simulink model "Vehicle_Model"  (R2022b)
settings: Solver=ode2  StartTime=T0  StopTime=Tf  FixedStep=Ts  EnableMultiTasking=on
model workspace (MAT data in the model file):
  aKalman : Simulink.Parameter (value not decoded)
  slipEnabler : Simulink.Parameter (value not decoded)
values from neighbouring files (symbols this model uses):
  enable_onlinePlots = 0    [main.m]
  enable_zoom = 1    [main.m]
  hv = 0.2    [main.m]
  lambda1_th = 0.1    [main.m]
  lambda2_th = 0.1    [main.m]
  LLC_sampleTime = LLC.sample_time    [main.m]
  longCTRparam = longitController()    [main.m]
  omega_LPF = 100    [main.m]
  previewPointParams = previewPointControllerParams()    [main.m]
  rho = 0.97    [main.m]
  rho_off = 0.9    [main.m]
  rho_on = 1.02    [main.m]
  road_data_sampled = [scenario_data.path.x_sampled', scenario_data.path.y_sampled']    [main.m]
  scenario_data = load(strcat('./Scenario/', scenario_name , '.mat'))    [main.m]
  T0 = scenario_data.times.t0    [main.m]
  tau_delta = vehicle_data.steering_system.tau_D    [main.m]
  Tb_dot_max = 5e3    (= 5000)    [main.m]
  Tb_max = 1000    [main.m]
  Tf = scenario_data.times.tf/2    [main.m]
  Ts = scenario_data.times.step_size    [main.m]
  v_on = 2.5    [main.m]
  v_stop = 0.1    [main.m]
  vehicle_data = getVehicleDataStruct()    [main.m]
  X0 = loadInitialConditions(scenario_data.vehicle_control.max_speed/3.6)    [main.m]
undefined symbols (not defined in the file or in its folder): DiscIntNeverNeededParam, latContr_select
libraries: simulink_extras x20, simulink x13, dspsigops x4, drivingvehiclecontroller x2, slpidlib x1
(part 2 of 2)

== system Vehicle_Model/Driver/Lateral Controller/Lateral Controller Clothoid-based ==
  targetPoint : Inport
  pose : Inport  Port=2
  speed : Inport  Port=3
  endOfCircuit : Inport  Port=4
  Action Port : ActionPort  ActionPortLabel=case [ 4 ]:
  MATLAB System : MATLABSystem  System=clothoidBased_lateralController  lookAhead=clothoidBasedParams.lookAhead  Kus=clothoidBasedParams.Kus  L=vehicle_data.vehicle.L  SimulateUsing=Interpreted execution
      mask Type: clothoidBased_lateralController
      mask Display:
      | disp('clothoidBased_lateralController');
      | port_label('input',1,'targetPoint');
      | port_label('input',2,'vehPose');
      | port_label('input',3,'vehSpeed');
      | port_label('input',4,'endOfCircuit');
      | port_label('output',1,'delta_req');
  Selector : Selector  InputPortWidth=4  IndexOptions=Index vector (dialog)  Indices=[1 2 3]  OutputSizes=1
  delta : Outport  VectorParamsAs1DForOutWhenUnconnected=off
  wires:
  speed/1 -> MATLAB System/3
  MATLAB System/1 -> delta/1
  pose/1 -> MATLAB System/2
  targetPoint/1 -> Selector/1
  Selector/1 -> MATLAB System/1
  endOfCircuit/1 -> MATLAB System/4

== system Vehicle_Model/Driver/Lateral Controller/Lateral Controller Stanley Dynamic ==
  targetPoint : Inport
  pose : Inport  Port=2
  speed : Inport  Port=3
  yaw_rate : Inport  Port=4
  steer_ang : Inport  Port=5
  Action Port : ActionPort  ActionPortLabel=case [ 3 ]:
  Constant : Constant
  Degrees to Radians : simulink_extras/Transformations/Degrees to Radians
  Helper Stanley Dynamic : MATLAB Function  TreatAsAtomicUnit=on
  Lateral Controller Stanley Dynamic : drivingvehiclecontroller/Lateral Controller Stanley  ModelType=Dynamic bicycle model  PositionGainF=stanleyParams.positGainFW  PositionGainR=stanleyParams.positGainREV  YawRateGain=stanleyParams.yawRateGain  DelayGain=stanleyParams.steerGain  VehicleMass=vehicle_data.vehicle.m  Lf=vehicle_data.vehicle.Lf  Lr=vehicle_data.vehicle.Lr  TireStiffness=stanleyParams.cornerStiff  Wheelbase=2.8  MaxSteeringAngle=stanleyParams.maxSteerAngle
  Radians to Degrees : simulink_extras/Transformations/Radians to Degrees
  Selector : Selector  InputPortWidth=4  IndexOptions=Index vector (dialog)  Indices=[1 2 3]  OutputSizes=1
  Selector1 : Selector  InputPortWidth=4  IndexOptions=Index vector (dialog)  Indices=[4]  OutputSizes=1
  delta : Outport  VectorParamsAs1DForOutWhenUnconnected=off
  wires:
  Lateral Controller Stanley Dynamic/1 -> Degrees to Radians/1
  pose/1 -> Helper Stanley Dynamic/1(pose)
  speed/1 -> Lateral Controller Stanley Dynamic/3
  Constant/1 -> Lateral Controller Stanley Dynamic/4
  Degrees to Radians/1 -> delta/1
  Helper Stanley Dynamic/1(currPose) -> Lateral Controller Stanley Dynamic/2
  targetPoint/1 -> Selector1/1, Selector/1
  Selector/1 -> Lateral Controller Stanley Dynamic/1
  Selector1/1 -> Lateral Controller Stanley Dynamic/5
  yaw_rate/1 -> Lateral Controller Stanley Dynamic/6
  Radians to Degrees/1 -> Lateral Controller Stanley Dynamic/7
  steer_ang/1 -> Radians to Degrees/1

== system Vehicle_Model/Driver/Lateral Controller/Lateral Controller Stanley Kinematic ==
  targetPoint : Inport
  pose : Inport  Port=2
  speed : Inport  Port=3
  Action Port : ActionPort  ActionPortLabel=case [ 2 ]:
  Constant : Constant
  Degrees to Radians : simulink_extras/Transformations/Degrees to Radians
  Helper Stanley Kinematic : MATLAB Function  TreatAsAtomicUnit=on
  Lateral Controller Stanley Kinematic : drivingvehiclecontroller/Lateral Controller Stanley  ModelType=Kinematic bicycle model  PositionGainF=stanleyParams.positGainFW  PositionGainR=stanleyParams.positGainREV  YawRateGain=0.2  DelayGain=0.2  VehicleMass=1575  Lf=1.2  Lr=1.6  TireStiffness=19000  Wheelbase=vehicle_data.vehicle.Lf + vehicle_data.vehicle.Lr  MaxSteeringAngle=stanleyParams.maxSteerAngle
  Selector : Selector  InputPortWidth=4  IndexOptions=Index vector (dialog)  Indices=[1 2 3]  OutputSizes=1
  delta : Outport  VectorParamsAs1DForOutWhenUnconnected=off
  wires:
  Lateral Controller Stanley Kinematic/1 -> Degrees to Radians/1
  pose/1 -> Helper Stanley Kinematic/1(pose)
  speed/1 -> Lateral Controller Stanley Kinematic/3
  Constant/1 -> Lateral Controller Stanley Kinematic/4
  Degrees to Radians/1 -> delta/1
  Helper Stanley Kinematic/1(currPose) -> Lateral Controller Stanley Kinematic/2
  targetPoint/1 -> Selector/1
  Selector/1 -> Lateral Controller Stanley Kinematic/1

== system Vehicle_Model/Driver/Lateral Controller/Preview point lateral Controller ==
  targetPoint : Inport
  endOfCircuit : Inport  Port=2
  Action Port : ActionPort  ActionPortLabel=case [ 5 ]:
  Constant : Constant  Value=previewPointParams.ke
  Constant1 : Constant  Value=previewPointParams.kp
  Preview Point Controller : MATLAB Function  TreatAsAtomicUnit=on
  delta : Outport  VectorParamsAs1DForOutWhenUnconnected=off
  wires:
  Preview Point Controller/1(delta) -> delta/1
  targetPoint/1 -> Preview Point Controller/1(target_Point)
  endOfCircuit/1 -> Preview Point Controller/4(endOfCircuit)
  Constant/1 -> Preview Point Controller/2(ke)
  Constant1/1 -> Preview Point Controller/3(kp)

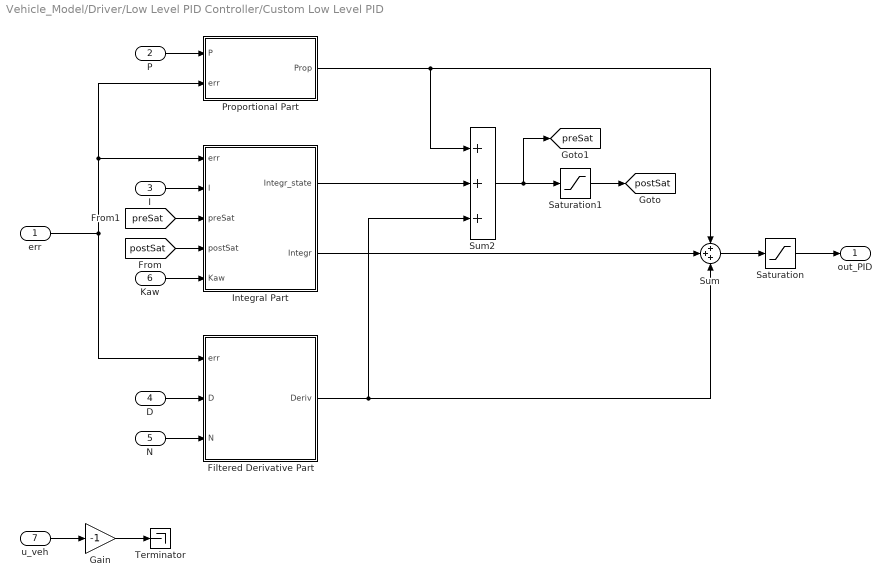
== system Vehicle_Model/Driver/Low Level PID Controller/Custom Low Level PID ==
  err : Inport
  P : Inport  Port=2
  I : Inport  Port=3
  D : Inport  Port=4
  N : Inport  Port=5
  Kaw : Inport  Port=6
  u_veh : Inport  Port=7
  Filtered Derivative Part : Subsystem
  Gain : Gain  Gain=-1
  Integral Part : Subsystem
  Proportional Part : Subsystem
  Saturation : Saturate  UpperLimit=1  LowerLimit=-1  LinearizeAsGain=off
  Saturation1 : Saturate  UpperLimit=1  LowerLimit=-1  LinearizeAsGain=off
  Sum : Sum  Inputs=+++
  Sum2 : Sum  Inputs=+++
  Terminator : Terminator
  out_PID : Outport  VectorParamsAs1DForOutWhenUnconnected=off
  tag scope: postSat=global, preSat=global
  wires:
  Sum2/1 -> [preSat], Saturation1/1
  Sum/1 -> Saturation/1
  Saturation/1 -> out_PID/1
  err/1 -> Filtered Derivative Part/1(err), Proportional Part/2(err), Integral Part/1(err)
  Saturation1/1 -> [postSat]
  I/1 -> Integral Part/2(I)
  Integral Part/1(Integr_state) -> Sum2/2
  Integral Part/2(Integr) -> Sum/2
  Proportional Part/1(Prop) -> Sum2/1, Sum/1
  P/1 -> Proportional Part/1(P)
  [preSat] -> Integral Part/3(preSat)
  [postSat] -> Integral Part/4(postSat)
  Filtered Derivative Part/1(Deriv) -> Sum/3, Sum2/3
  D/1 -> Filtered Derivative Part/2(D)
  N/1 -> Filtered Derivative Part/3(N)
  u_veh/1 -> Gain/1
  Gain/1 -> Terminator/1
  Kaw/1 -> Integral Part/5(Kaw)

== system Vehicle_Model/Driver/Low Level PID Controller/Custom Low Level PID/Filtered Derivative Part ==
  err : Inport
  D : Inport  Port=2
  N : Inport  Port=3
  Constant : Constant
  Discrete Transfer Fcn : DiscreteTransferFcn  Numerator=[1 -1]  DenominatorSource=Input port  SampleTime=Ts  a0EqualsOne=on
      settings: InputPortMap=u0,p3
  Gain1 : Gain  Gain=Ts/2
  Math Function : Math  Operator=reciprocal  SignedPower=on
  Mux1 : Mux  Inputs=2
  Product{2..5} (4 alike) : Product
  SumDen : Sum  Inputs=++|
  SumNum : Sum  Inputs=-+|
  Deriv : Outport  VectorParamsAs1DForOutWhenUnconnected=off
  wires:
  N/1 -> Gain1/1, Product5/2
  Product4/1 -> Product5/1
  SumDen/1 -> Math Function/1
  Math Function/1 -> Product4/2, Product3/1
  SumNum/1 -> Product3/2
  Product2/1 -> Discrete Transfer Fcn/1
  Discrete Transfer Fcn/1 -> Product4/1
  Constant/1 -> SumNum/1, SumDen/1, Mux1/1
  Product3/1 -> Mux1/2
  Mux1/1 -> Discrete Transfer Fcn/2
  Gain1/1 -> SumNum/2, SumDen/2
  err/1 -> Product2/1
  D/1 -> Product2/2
  Product5/1 -> Deriv/1

== system Vehicle_Model/Driver/Low Level PID Controller/Custom Low Level PID/Integral Part ==
  err : Inport
  I : Inport  Port=2
  preSat : Inport  Port=3
  postSat : Inport  Port=4
  Kaw : Inport  Port=5
  Anti-windup : Subsystem
  Discrete-Time Integrator1 : DiscreteIntegrator  IntegratorMethod=Integration: Trapezoidal  SampleTime=Ts  ShowStatePort=on  ICPrevOutput=DiscIntNeverNeededParam  ICPrevScaledInput=DiscIntNeverNeededParam
  Product1 : Product
  Integr_state : Outport  VectorParamsAs1DForOutWhenUnconnected=off
  Integr : Outport  Port=2  VectorParamsAs1DForOutWhenUnconnected=off
  wires:
  Discrete-Time Integrator1/State -> Integr_state/1
  preSat/1 -> Anti-windup/2(preSat)
  Product1/1 -> Anti-windup/4(preInt)
  postSat/1 -> Anti-windup/3(postSat)
  I/1 -> Product1/2
  Anti-windup/1(Out_antiWindUp) -> Discrete-Time Integrator1/1
  Discrete-Time Integrator1/1 -> Integr/1
  err/1 -> Product1/1
  Kaw/1 -> Anti-windup/1(Kaw)

== system Vehicle_Model/Driver/Low Level PID Controller/Custom Low Level PID/Proportional Part ==
  P : Inport
  err : Inport  Port=2
  Product : Product
  Prop : Outport  VectorParamsAs1DForOutWhenUnconnected=off
  wires:
  P/1 -> Product/2
  Product/1 -> Prop/1
  err/1 -> Product/1

== system Vehicle_Model/Driver/Low Level PID Controller/Custom Low Level PID/Integral Part/Anti-windup ==
  Kaw : Inport
  preSat : Inport  Port=2
  postSat : Inport  Port=3
  preInt : Inport  Port=4
  Product : Product
  Sum : Sum  Inputs=|-+
  Sum1 : Sum  Inputs=|++
  Out_antiWindUp : Outport  VectorParamsAs1DForOutWhenUnconnected=off
  wires:
  preSat/1 -> Sum/1
  preInt/1 -> Sum1/2
  Product/1 -> Sum1/1
  Sum1/1 -> Out_antiWindUp/1
  Sum/1 -> Product/2
  postSat/1 -> Sum/2
  Kaw/1 -> Product/1

== matlab function Vehicle_Model/Vehicle Model ==
  settings: sampleTime=step_size
  data: dX_prev input; X input; Tw__rr_brake input; Tw__rl_brake input; Tw__fr_brake input; Tw__fl_brake input; Tm_req input; dX output; extra_params output; delta_req input; vehicle_data parameter; road_condition input
function [dX,extra_params] = Vehicle_model(dX_prev,X,Tw__rr_brake,Tw__rl_brake,Tw__fr_brake,Tw__fl_brake,Tm_req,delta_req,vehicle_data,road_condition)

% ----------------------------------------------------------------
%% Double Track Vehicle Model
%  authors: 
%  rev. 1.0 Mattia Piccinini & Gastone Pietro Papini Rosati
%  rev. 2.0 Edoardo Pagot
%  date:
%  rev 1.0:    13/10/2020
%  rev 2.0:    16/05/2022
% ----------------------------------------------------------------


% ----------------------------------------------------------------
%% INPUTS OF THE MODEL
% ----------------------------------------------------------------

% Model inputs are: 
%       - requested wheel torques
%       - requested steering angle at the steering wheel delta_req (in [rad])


% ----------------------------------------------------------------
%% OUTPUTS OF THE MODEL
% ----------------------------------------------------------------

% The outputs of the model are the derivatives of all vehicle states,
% collected in the dX vector, as well as some other useful extra parameters 
% to describe vehicle behavior, saved in the extra_params vector

% Empty output vectors are here initialized 
dX = zeros(23,1);  
extra_params = zeros(23,1);  


% ----------------------------------------------------------------
%% STATES OF THE MODEL
% ----------------------------------------------------------------

x         = X(1);       % [m] x-coord of the vehicle CoM
y         = X(2);       % [m] x-coord of the vehicle CoM
psi       = X(3);       % [rad] yaw angle
u         = X(4);       % [m/s] vehicle longitudinal speed
v         = X(5);       % [m/s] vehicle lateral speed
Omega     = X(6);       % [rad/s] yaw rate
Fz__rr    = X(7);       % [N] vertical force for the rear right wheel
Fz__rl    = X(8);       % [N] vertical force for the rear left wheel
Fz__fr    = X(9);       % [N] vertical force for the front right wheel
Fz__fl    = X(10);      % [N] vertical force for the front left wheel
delta     = X(11);      % [rad] steering angle (at the wheel)
omega__rr = X(12);      % [rad/s] rotational speed rear right wheel
omega__rl = X(13);      % [rad/s] rotational speed rear left wheel 
omega__fr = X(14);      % [rad/s] rotational speed front right wheel 
omega__fl = X(15);      % [rad/s] rotational speed front left wheel 
alpha__rr = X(16);      % [rad] side slip angle rear right wheel
alpha__rl = X(17);      % [rad] side slip angle rear left wheel
alpha__fr = X(18);      % [rad] side slip angle front right wheel
alpha__fl = X(19);      % [rad] side slip angle front left wheel
kappa__rr = X(20);      % [-] longitudinal slip rear right wheel
kappa__rl = X(21);      % [-] longitudinal slip rear left wheel
kappa__fr = X(22);      % [-] longitudinal slip front right wheel
kappa__fl = X(23);      % [-] longitudinal slip front left wheel

% ----------------------------------------------------------------
%% AUXILIARY MODELS
% ----------------------------------------------------------------

% ----------------------
% MOTOR MODEL
% ----------------------
% Driving torques at the wheels
Tw__rr_traction = MotorModel(Tm_req,omega__rr,vehicle_data);
Tw__rl_traction = MotorModel(Tm_req,omega__rl,vehicle_data);

% Rear wheels braking model
Tw__rr_brake = brakeModelRear(Tw__rr_brake,omega__rr,vehicle_data); 
Tw__rl_brake = brakeModelRear(Tw__rl_brake,omega__rl,vehicle_data); 
% Front wheels braking model
Tw__fr_brake = brakeModelFront(Tw__fr_brake,omega__fr,vehicle_data);
Tw__fl_brake = brakeModelFront(Tw__fl_brake,omega__fl,vehicle_data);

% Total Torques
Tw__rr = Tw__rr_brake + Tw__rr_traction;
Tw__rl = Tw__rl_brake + Tw__rl_traction;
Tw__fr = Tw__fr_brake;
Tw__fl = Tw__fl_brake;


% ----------------------
% CAMBER MODEL
% ----------------------
[gamma__rr, gamma__rl, gamma__fr, gamma__fl] = camberModel(vehicle_data);

% ----------------------
% ACKERMANN STEERING MODEL
% ----------------------
% Compute steering angles for front wheels, with perfect Ackerman steering model
[delta__fr, delta__fl] = perfectAcker(delta,vehicle_data);

% ----------------------
% AERODYNAMIC MODEL
% ----------------------
% Aero drag, downforce at rear axle, downforce at front axle
[FAxc, FAz__r, FAz__f] = aeroModel(u,vehicle_data);

% ----------------------
% LONGITUDINAL SLIPS
% ----------------------
% Longitudinal slip model including a correction for low speed 
[kappa__rr_corr,kappa__rl_corr,kappa__fr_corr,kappa__fl_corr] = long_slip_low_speed(u,Omega,kappa__rr,kappa__rl,kappa__fr,kappa__fl,omega__rr,omega__rl,omega__fr,omega__fl,delta__fr,delta__fl,Fz__rr,Fz__rl,Fz__fr,Fz__fl,gamma__rr,gamma__rl,gamma__fr,gamma__fl,vehicle_data, road_condition);
          
% ----------------------
% ROAD CONDITION
% ----------------------
% Compute the aderenace of the asphalt 
road_condition_rr = road_condition(1);
road_condition_rl = road_condition(2);
road_condition_fr = road_condition(3);
road_condition_fl = road_condition(4);

% ----------------------
% TIRE PACEJKA MODEL
% ----------------------
% Ensure symmetric behavior of left and right tires by calculating the
% forces and moments for left tires via a previous change of sign of the
% side slip alpha and the camber gamma
% Side slip sign must be changed since data were fitted with reverse alpha
% sign

% RR
Fx__rr =  MF96_FX(kappa__rr_corr, -alpha__rr, -gamma__rr, Fz__rr, vehicle_data.tyre_data_r, road_condition_rr);
Fy__rr = -MF96_FY(kappa__rr_corr,  alpha__rr, -gamma__rr, Fz__rr, vehicle_data.tyre_data_r, road_condition_rr); % mirrored
AM__rr = -MF96_MZ(kappa__rr_corr,  alpha__rr, -gamma__rr, Fz__rr, vehicle_data.tyre_data_r, road_condition_rr); % mirrored

% RL
Fx__rl = MF96_FX(kappa__rl_corr, -alpha__rl, gamma__rl, Fz__rl, vehicle_data.tyre_data_r, road_condition_rl);
Fy__rl = MF96_FY(kappa__rl_corr, -alpha__rl, gamma__rl, Fz__rl, vehicle_data.tyre_data_r, road_condition_rl);
AM__rl = MF96_MZ(kappa__rl_corr, -alpha__rl, gamma__rl, Fz__rl, vehicle_data.tyre_data_r, road_condition_rl);

%FR
Fx__fr =  MF96_FX(kappa__fr_corr, -alpha__fr, -gamma__fr, Fz__fr, vehicle_data.tyre_data_f, road_condition_fr);
Fy__fr = -MF96_FY(kappa__fr_corr,  alpha__fr, -gamma__fr, Fz__fr, vehicle_data.tyre_data_f, road_condition_fr); % mirrored
AM__fr = -MF96_MZ(kappa__fr_corr,  alpha__fr, -gamma__fr, Fz__fr, vehicle_data.tyre_data_f, road_condition_fr); % mirrored

% FL
Fx__fl = MF96_FX(kappa__fl_corr, -alpha__fl, gamma__fl, Fz__fl, vehicle_data.tyre_data_f, road_condition_fl);
Fy__fl = MF96_FY(kappa__fl_corr, -alpha__fl, gamma__fl, Fz__fl, vehicle_data.tyre_data_f, road_condition_fl);
AM__fl = MF96_MZ(kappa__fl_corr, -alpha__fl, gamma__fl, Fz__fl, vehicle_data.tyre_data_f, road_condition_fl);


Mz_tires.rr = AM__rr;  Mz_tires.rl = AM__rl;  Mz_tires.fr = AM__fr;  Mz_tires.fl = AM__fl;

% ----------------------
% VERTICAL TIRE FORCES MODEL
% ----------------------
% Compute vertical tire loads
u_dot = dX_prev(4);
VerticalForces = LoadTransferModel(Omega,u,u_dot,FAz__r,FAz__f,Mz_tires,vehicle_data);
Fz__rr__ss = VerticalForces.Fz_rr_ss;
Fz__rl__ss = VerticalForces.Fz_rl_ss;
Fz__fr__ss = VerticalForces.Fz_fr_ss;
Fz__fl__ss = VerticalForces.Fz_fl_ss;

% ----------------------
% AXLE FORCES
% ----------------------
Fx__r = Fx__rr + Fx__rl;
Fx__f = Fx__fl - sin(delta__fl)*Fy__fl + Fx__fr - sin(delta__fr)*Fy__fr;
Fy__r = Fy__rl + Fy__rr;
Fy__f = sin(delta__fl)*Fx__fl + Fy__fl + sin(delta__fr)*Fx__fr + Fy__fr;
Delta__Fx__r = (Fx__rr-Fx__rl)/2;
Delta__Fx__f = ((Fx__fr - sin(delta__fr)*Fy__fr) - (Fx__fl - sin(delta__fl)*Fy__fl))/2;


% ----------------------
% STEADY STATE SLIPS
% ----------------------
% Longitudinal Slips
[kappa__rr__ss,kappa__rl__ss,kappa__fr__ss,kappa__fl__ss] = steadyStateLongSlips(omega__rr,omega__rl,omega__fr,omega__fl,Omega,u,delta__fr,delta__fl,vehicle_data);
% Lateral Slips
[alpha__rr__ss,alpha__rl__ss,alpha__fr__ss,alpha__fl__ss] = steadyStateLatSlips(Omega,u,v,delta__fr,delta__fl,vehicle_data);


% ----------------------------------------------------------------
%% VEHICLE DATA
% ----------------------------------------------------------------
m      = vehicle_data.vehicle.m;
Lf     = vehicle_data.vehicle.Lf;
Lr     = vehicle_data.vehicle.Lr;
Wf     = vehicle_data.vehicle.Wf;
Wr     = vehicle_data.vehicle.Wr;
izz    = vehicle_data.vehicle.i_zz;
tau__N = vehicle_data.suspension.tau_N;
tau__D = vehicle_data.steering_system.tau_D;
tau__H = vehicle_data.steering_system.tau_H;
ly     = vehicle_data.vehicle.ly;
lx     = vehicle_data.vehicle.lx;
iwa__r = vehicle_data.rear_wheel.iwa_r;
iwa__f = vehicle_data.front_wheel.iwa_f;
Rr     = vehicle_data.rear_wheel.Rr;
Rf     = vehicle_data.front_wheel.Rf;

% ----------------------------------------------------------------
%% VEHICLE MODEL DIFFERENTIAL EQUATIONS
% ----------------------------------------------------------------

% The following system of ODE is imported from Maple symbolic model

% Evolution of vehicle pose
x_dot        = u*cos(psi) - v*sin(psi);
y_dot        = v*cos(psi) + u*sin(psi);
psi_dot      = Omega;
% Newton equations
u_Dot        = (Omega * m * v - FAxc + Fx__f + Fx__r) / m;
v_Dot        = (-Omega * m * u + Fy__f + Fy__r) / m;
% Euler equation
Omega_Dot    = (Lf * Fy__f - Lr * Fy__r + Wf * Delta__Fx__f + Wr * Delta__Fx__r + AM__fl + AM__fr + AM__rl + AM__rr) / izz;
% Vertical loads first order dynamics
Fz_rr_Dot    = (-Fz__rr + Fz__rr__ss) / tau__N;
Fz_rl_Dot    = (-Fz__rl + Fz__rl__ss) / tau__N;
Fz_fr_Dot    = (-Fz__fr + Fz__fr__ss) / tau__N;
Fz_fl_Dot    = (-Fz__fl + Fz__fl__ss) / tau__N;
% Steering wheel first order dynamics
delta_Dot    = (-delta * tau__D + delta_req) / tau__D / tau__H;
% Side slip angle first order dynamics
alpha_rr_Dot = -(alpha__rr - alpha__rr__ss) * abs(u) / ly;
alpha_rl_Dot = -(alpha__rl - alpha__rl__ss) * abs(u) / ly;
alpha_fr_Dot = -(alpha__fr - alpha__fr__ss) * abs(u) / ly;
alpha_fl_Dot = -(alpha__fl - alpha__fl__ss) * abs(u) / ly;
% Longitudinal slip first order dynamics
kappa_rr_Dot = -abs(u) * (kappa__rr - kappa__rr__ss) / lx;
kappa_rl_Dot = -abs(u) * (kappa__rl - kappa__rl__ss) / lx;
kappa_fr_Dot = -abs(u) * (kappa__fr - kappa__fr__ss) / lx;
kappa_fl_Dot = -abs(u) * (kappa__fl - kappa__fl__ss) / lx;
% Wheel spin dynamics
omega_rr_Dot = (-Fx__rr * Rr + Tw__rr) / iwa__r;
omega_rl_Dot = (-Fx__rl * Rr + Tw__rl) / iwa__r;
omega_fr_Dot = (-Fx__fr * Rf + Tw__fr) / iwa__f;
omega_fl_Dot = (-Fx__fl * Rf + Tw__fl) / iwa__f;

% Collect states derivatives in the dX vector
dX(1)  = x_dot;
dX(2)  = y_dot;
dX(3)  = psi_dot;
dX(4)  = u_Dot;
dX(5)  = v_Dot;
dX(6)  = Omega_Dot;
dX(7)  = Fz_rr_Dot;
dX(8)  = Fz_rl_Dot;
dX(9)  = Fz_fr_Dot;
dX(10) = Fz_fl_Dot;
dX(11) = delta_Dot;
dX(12) = omega_rr_Dot;
dX(13) = omega_rl_Dot;
dX(14) = omega_fr_Dot;
dX(15) = omega_fl_Dot;
dX(16) = alpha_rr_Dot;
dX(17) = alpha_rl_Dot;
dX(18) = alpha_fr_Dot;
dX(19) = alpha_fl_Dot;
dX(20) = kappa_rr_Dot;
dX(21) = kappa_rl_Dot;
dX(22) = kappa_fr_Dot;
dX(23) = kappa_fl_Dot;


% ----------------------------------------------------------------
%% SAVE USEFUL EXTRA PARAMETERS
% ----------------------------------------------------------------

extra_params(1)  = Tw__rr;
extra_params(2)  = Tw__rl;
extra_params(3)  = Tw__fr;
extra_params(4)  = Tw__fl;
extra_params(5)  = Fx__rr;
extra_params(6)  = Fx__rl;
extra_params(7)  = Fx__fr;
extra_params(8)  = Fx__fl;
extra_params(9)  = Fy__rr;
extra_params(10) = Fy__rl;
extra_params(11) = Fy__fr;
extra_params(12) = Fy__fl;
extra_params(13) = AM__rr;
extra_params(14) = AM__rl;
extra_params(15) = AM__fr;
extra_params(16) = AM__fl;
extra_params(17) = gamma__rr;
extra_params(18) = gamma__rl;
extra_params(19) = gamma__fr;
extra_params(20) = gamma__fl;
extra_params(21) = delta__fr;
extra_params(22) = delta__fl;
extra_params(23) = delta_req;

end

== matlab function Vehicle_Model/ABS and Wheel torque generation/ABS Rear Right Wheel1/compute lambda ==
  data: u input; lambda output; omega input; vehicle_data parameter
function lambda = compute_lambda(u, omega, vehicle_data)

lambda = (u - omega*vehicle_data.rear_wheel.Rr)/u;

== stateflow chart Vehicle_Model/ABS and Wheel torque generation/ABS Rear Left Wheel1/Antilock Braking System/Activation and Deactivation Logic ==
  state abs_OFF
    ABS_ON = 0;
    state High_Speed_OFF
      Tb_select = 1;
    state Low_Speed_OFF
      Tb_select = 1;
    (default) -> High_Speed_OFF
    High_Speed_OFF -> Low_Speed_OFF [order 2] : [v < v_on - hv]
    Low_Speed_OFF -> High_Speed_OFF : [v > v_on + hv]
  state abs_ON
    ABS_ON = 1;
    state High_Speed_ON
      Tb_select = 2;
    state Low_Speed_ON
      Tb_select = 3;
    High_Speed_ON -> Low_Speed_ON [order 2] : [v < v_on]
  (default) -> abs_OFF
  High_Speed_OFF -> High_Speed_ON [order 1] : [v > v_on && ...
      | Tb_Dr > rho_on * Tb_Ctrl && ...
      | lambda > lambda1_th - (((lambda1_th - lambda2_th) * Tb_dot) / Tb_dot_max) ]
  High_Speed_ON -> High_Speed_OFF [order 1] : [Tb_Dr < rho_off * Tb_Ctrl]
  Low_Speed_ON -> Low_Speed_OFF : [v < v_stop || ...
      | Tb_Dr < rho_off * Tb_LPF]
  data: Tb_select output; Tb_Dr input; Tb_Ctrl input; v input; Tb_dot input; Tb_dot_max parameter; v_on parameter; rho_on parameter; Tb_LPF input; lambda input; lambda1_th parameter; v_stop parameter; hv parameter; rho_off parameter; ABS_ON output; lambda2_th parameter

== matlab function Vehicle_Model/ABS and Wheel torque generation/ABS Rear Left Wheel1/compute lambda ==
  data: u input; lambda output; omega input; vehicle_data parameter
function lambda = compute_lambda(u, omega, vehicle_data)

lambda = (u - omega*vehicle_data.rear_wheel.Rr)/u;

== stateflow chart Vehicle_Model/ABS and Wheel torque generation/ABS Front Right Wheel1/Antilock Braking System/Activation and Deactivation Logic ==
  state abs_OFF
    ABS_ON = 0;
    state High_Speed_OFF
      Tb_select = 1;
    state Low_Speed_OFF
      Tb_select = 1;
    (default) -> High_Speed_OFF
    High_Speed_OFF -> Low_Speed_OFF [order 2] : [v < v_on - hv]
    Low_Speed_OFF -> High_Speed_OFF : [v > v_on + hv]
  state abs_ON
    ABS_ON = 1;
    state High_Speed_ON
      Tb_select = 2;
    state Low_Speed_ON
      Tb_select = 3;
    High_Speed_ON -> Low_Speed_ON [order 2] : [v < v_on]
  (default) -> abs_OFF
  High_Speed_OFF -> High_Speed_ON [order 1] : [v > v_on && ...
      | Tb_Dr > rho_on * Tb_Ctrl && ...
      | lambda > lambda1_th - (((lambda1_th - lambda2_th) * Tb_dot) / Tb_dot_max) ]
  High_Speed_ON -> High_Speed_OFF [order 1] : [Tb_Dr < rho_off * Tb_Ctrl]
  Low_Speed_ON -> Low_Speed_OFF : [v < v_stop || ...
      | Tb_Dr < rho_off * Tb_LPF]
  data: Tb_select output; Tb_Dr input; Tb_Ctrl input; v input; Tb_dot input; Tb_dot_max parameter; v_on parameter; rho_on parameter; Tb_LPF input; lambda input; lambda1_th parameter; v_stop parameter; hv parameter; rho_off parameter; ABS_ON output; lambda2_th parameter

== matlab function Vehicle_Model/ABS and Wheel torque generation/ABS Front Right Wheel1/compute lambda ==
  data: u input; lambda output; omega input; vehicle_data parameter
function lambda = compute_lambda(u, omega, vehicle_data)

lambda = (u - omega*vehicle_data.rear_wheel.Rr)/u;

== matlab function Vehicle_Model/Estimate pose/Online Trajectory Plots/Plot manager ==
  data: vehiclePose input; targetPoint_steerCtrl input; enable_zoomMPC input; refPath input; latContr_type input
function real_time_plot(vehiclePose,targetPoint_steerCtrl,enable_zoomMPC,refPath,latContr_type)
    
    coder.extrinsic('patch');
    
    %% Extract vehicle pose
    xCoMCar = vehiclePose(1);
    yCoMCar = vehiclePose(2);
    vehicleAttitude = vehiclePose(3);
    
    %% Load vehicle data
    vehicle_data = getVehicleDataStruct();
    Lf = vehicle_data.vehicle.Lf;        
    Lr = vehicle_data.vehicle.Lr;                 
    Wf = vehicle_data.vehicle.Wf;     
    Wr = vehicle_data.vehicle.Wr;
    
    %% Delete the plots for the previous iteration
    cla;
    
    %% Sketch the vehicle and its position, for this MPC iteration
    % Rotation matrix from vehicle (mobile) frame to the absolute frame
    RotMat = [cos(vehicleAttitude), -sin(vehicleAttitude); ...
              sin(vehicleAttitude), cos(vehicleAttitude)];
    
    pos_vehRR = RotMat*[-Lr -Wr/2]';
    pos_vehRL = RotMat*[-Lr +Wr/2]';
    pos_vehFR = RotMat*[+Lf -Wf/2]';
    pos_vehFL = RotMat*[+Lf +Wf/2]';
    pos_veh   = [pos_vehRR pos_vehRL pos_vehFL pos_vehFR];
    
    % Optimal route computed with route planner
    X_route = refPath(:,1);
    Y_route = refPath(:,2);
    plot(X_route,Y_route,'go','MarkerSize',2)
    
    % Current vehicle pose
    patch(xCoMCar + pos_veh(1,:),yCoMCar + pos_veh(2,:),'yellow');
    
    % Objects of the road scenario (walls, fixed obstacles etc)
%     for ii=1:size(mapObjects,1)
%         rectangle('Position',mapObjects(ii,:),'FaceColor',color('purple'),'EdgeColor',color('purple'),'LineWidth',2)
%     end
    
    % Target point used by some low-level lateral controllers
    if (latContr_type==1 || latContr_type==4)  
        plot(targetPoint_steerCtrl(1),targetPoint_steerCtrl(2),'r*','MarkerSize',6)
    end
    
    % Zoom on the vehicle if required
    if (enable_zoomMPC)
        xlim([xCoMCar-40 xCoMCar+40])
        ylim([yCoMCar-40 yCoMCar+40])
    end
    
end

== stateflow chart Vehicle_Model/ABS and Wheel torque generation/ABS Front Left Wheel1/Antilock Braking System/Activation and Deactivation Logic ==
  state abs_OFF
    ABS_ON = 0;
    state High_Speed_OFF
      Tb_select = 1;
    state Low_Speed_OFF
      Tb_select = 1;
    (default) -> High_Speed_OFF
    High_Speed_OFF -> Low_Speed_OFF [order 2] : [v < v_on - hv]
    Low_Speed_OFF -> High_Speed_OFF : [v > v_on + hv]
  state abs_ON
    ABS_ON = 1;
    state High_Speed_ON
      Tb_select = 2;
    state Low_Speed_ON
      Tb_select = 3;
    High_Speed_ON -> Low_Speed_ON [order 2] : [v < v_on]
  (default) -> abs_OFF
  High_Speed_OFF -> High_Speed_ON [order 1] : [v > v_on && ...
      | Tb_Dr > rho_on * Tb_Ctrl && ...
      | lambda > lambda1_th - (((lambda1_th - lambda2_th) * Tb_dot) / Tb_dot_max) ]
  High_Speed_ON -> High_Speed_OFF [order 1] : [Tb_Dr < rho_off * Tb_Ctrl]
  Low_Speed_ON -> Low_Speed_OFF : [v < v_stop || ...
      | Tb_Dr < rho_off * Tb_LPF]
  data: Tb_select output; Tb_Dr input; Tb_Ctrl input; v input; Tb_dot input; Tb_dot_max parameter; v_on parameter; rho_on parameter; Tb_LPF input; lambda input; lambda1_th parameter; v_stop parameter; hv parameter; rho_off parameter; ABS_ON output; lambda2_th parameter

== stateflow chart Vehicle_Model/ABS and Wheel torque generation/ESP/Braking logic ==
  state ESP_ON
    state Brake_front
      state Front_left
        gain = [-1,0,0,0];
      state Front_right
        gain = [0,1,0,0];
      (default) -> Front_left
      (junction 30) -> Front_left [order 1] : [omega < 0]
      (junction 30) -> Front_right [order 2] : [omega > 0]
    state Brake_rear
      state Rear_left
        gain = [0,0,-1,0];
      state Rear_right
        gain = [0,0,0,1];
      (junction 34) -> Rear_left [order 2] : [omega > 0]
      (junction 34) -> Rear_right [order 1] : [omega < 0]
    (default) -> Brake_front
    Brake_rear -> (junction 25) : [err_omega < 0]
    (junction 25) -> (junction 30) [order 2] : [err_omega < 0]
    (junction 25) -> (junction 34) [order 1] : [err_omega > 0]
    Brake_front -> (junction 25) : [err_omega > 0]
  state ESP_OFF
    gain = [0,0,0,0];
  (default) -> ESP_ON
  ESP_OFF -> (junction 25) : [abs(err_omega) > max_omega_err + 0.01]
  ESP_ON -> ESP_OFF : [abs(err_omega)  < max_omega_err - 0.01]
  data: err_omega input; omega input; max_omega_err input; gain output

== matlab function Vehicle_Model/MATLAB Function ==
  data: start input; stop input; step input; idx input
% progress_bar is a simple utility developed to easily incorporate a progress
% bar in any MATLAB loop.
%
% Authors
% -------
%  - Sebastiano Taddei.
%
function progress_bar(start, stop, step, idx)
%PROGRESS_BAR
%   Prints a progress bar to the console.
%
%   Arguments
%   ---------
%    - start -> start index.
%    - stop  -> stop index.
%    - step  -> step to take.
%    - idx   -> current index.
%    - type  -> the type of progress bar:
%                - 0 -> XXX%;
%                - 1 -> [===    ].
%

coder.extrinsic('fprintf');

last = floor( (stop - start) / step ) * step + start;
perc = floor( idx / (last - start) * 100 );

if idx ~= start
    fprintf('\b\b\b\b\b%3d%%\n', perc);
else
    fprintf('%3d%%\n', perc);
end

end

== matlab function Vehicle_Model/ABS and Wheel torque generation/ABS Front Left Wheel1/compute lambda ==
  data: u input; lambda output; omega input; vehicle_data parameter
function lambda = compute_lambda(u, omega, vehicle_data)

lambda = (u - omega*vehicle_data.rear_wheel.Rr)/u;

== matlab function Vehicle_Model/Driver/Lateral Controller/Preview point lateral Controller/Preview Point Controller ==
  data: target_Point input; delta output; ke input; kp input; endOfCircuit input
function delta  = previewPoint(target_Point,ke,kp,endOfCircuit)

    delta = target_Point(1) * ke + target_Point(3) * kp;
   
end

== matlab function Vehicle_Model/Driver/Lateral Controller/Arc Path Following Controller/Arc Path Following Controller ==
  data: target_Point input; delta output; pose input; endOfCircuit input
function delta  = arcPathFollowController(target_Point,pose,endOfCircuit)

    % Load vehicle params
    vehicle_params = getVehicleDataStruct();
    Lf = vehicle_params.vehicle.Lf;        
    Lr = vehicle_params.vehicle.Lr;    
    L  = Lf + Lr;  % [m] vehicle wheelbase
    
    % Current vehicle center of mass pose 
    x_C     = pose(1);
    y_C     = pose(2);
    theta_C = pose(3);  % vehicle attitude (in radians)
     
    % Rotation matrix from vehicle frame to absolute frame
    Rot_mat = [cos(theta_C), -sin(theta_C); ...
               sin(theta_C),  cos(theta_C)];
    
    % Point of the vehicle in correspondence with the rear axle
    x_R = x_C - Lr*cos(theta_C);
    y_R = y_C - Lr*sin(theta_C);
    current_point = [x_R y_R];
    
    % Express the current_point in the vehicle frame
    current_point_vehFrame = [-Lr,0];
    
    % Distance from the current position to the target point
    distFromTarget = sqrt((target_Point(1)-current_point(1))^2 + (target_Point(2)-current_point(2))^2);
    
    % Express the target_Point in the vehicle frame
    target_Point_vehFrame = Rot_mat'*(target_Point(1:2)' - current_point');
    
    % Angle measured w.r.t. the vehicle reference frame
    gamma = atan2((target_Point_vehFrame(2)-current_point_vehFrame(2))/distFromTarget,(target_Point_vehFrame(1)-current_point_vehFrame(1))/distFromTarget);
    
    % Required curvature radius
    R = 0.5*distFromTarget/sin(gamma);
   
    if (~endOfCircuit)
        delta = atan(L/R);    
    else
        delta = 0;
    end

end

== matlab function Vehicle_Model/ABS and Wheel torque generation/Powertrain ==
  data: ped input; vehicle_data parameter; Tw__rr_brake output; Tw__rl_brake output; Tw__fr_brake output; Tw__fl_brake output; Tm_req output
function [Tw__rr_brake,Tw__rl_brake,Tw__fr_brake,Tw__fl_brake,Tm_req] = powertrain(ped, vehicle_data)

% ----------------------
% MOTOR MODEL
% ----------------------
% Driving torques at the wheels
Tm_req = posPart(ped)*vehicle_data.motor.maxTorque;
 
% ----------------------
% BRAKE MODEL
% ----------------------
Tb_r_req = -negPart(ped)*vehicle_data.braking.totBrakeTorque*(1-vehicle_data.braking.brakeRatio);
Tb_f_req = -negPart(ped)*vehicle_data.braking.totBrakeTorque*vehicle_data.braking.brakeRatio;


% Rear wheels braking model
Tw__rr_brake = Tb_r_req; 
Tw__rl_brake = Tb_r_req; 
% Front wheels braking model
Tw__fr_brake = Tb_f_req; 
Tw__fl_brake = Tb_f_req; 


end

== matlab function Vehicle_Model/Driver/Lateral Controller/Lateral Controller Stanley Dynamic/Helper Stanley Dynamic ==
  data: pose input; currPose output
function currPose = helperStanleyDyn(pose)

    currPose = [pose(1), pose(2), rad2deg(pose(3))];

end

== matlab function Vehicle_Model/Subsystem1/MATLAB Function ==
  data: x input; a_x input; x_dot output size=2; a_y input; omega input; u_meas input; gamma input
function x_dot   = kine_observer(x, a_x, a_y, omega, u_meas, gamma)

A = [   0    omega;
     -omega    0];

B = [1 0;
     0 1];

u = [a_x;
     a_y];

C = [1 0];

L = [2*gamma*abs(omega);
     (gamma^2 - 1)*omega];

x_dot = (A - L*C)*x + B*u + L*u_meas;

== matlab function Vehicle_Model/Driver/Lateral Controller/Lateral Controller Stanley Kinematic/Helper Stanley Kinematic ==
  data: pose input; currPose output
function currPose = helperStanleyKine(pose)

    currPose = [pose(1), pose(2), rad2deg(pose(3))];

end

== stateflow chart Vehicle_Model/ABS and Wheel torque generation/ABS Rear Right Wheel1/Antilock Braking System/Activation and Deactivation Logic ==
  state abs_OFF
    ABS_ON = 0;
    state High_Speed_OFF
      Tb_select = 1;
    state Low_Speed_OFF
      Tb_select = 1;
    (default) -> High_Speed_OFF
    High_Speed_OFF -> Low_Speed_OFF [order 2] : [v < v_on - hv]
    Low_Speed_OFF -> High_Speed_OFF : [v > v_on + hv]
  state abs_ON
    ABS_ON = 1;
    state High_Speed_ON
      Tb_select = 2;
    state Low_Speed_ON
      Tb_select = 3;
    High_Speed_ON -> Low_Speed_ON [order 2] : [v < v_on]
  (default) -> abs_OFF
  High_Speed_OFF -> High_Speed_ON [order 1] : [v > v_on && ...
      | Tb_Dr > rho_on * Tb_Ctrl && ...
      | lambda > lambda1_th - (((lambda1_th - lambda2_th) * Tb_dot) / Tb_dot_max) ]
  High_Speed_ON -> High_Speed_OFF [order 1] : [Tb_Dr < rho_off * Tb_Ctrl]
  Low_Speed_ON -> Low_Speed_OFF : [v < v_stop || ...
      | Tb_Dr < rho_off * Tb_LPF]
  data: Tb_select output; Tb_Dr input; Tb_Ctrl input; v input; Tb_dot input; Tb_dot_max parameter; v_on parameter; rho_on parameter; Tb_LPF input; lambda input; lambda1_th parameter; v_stop parameter; hv parameter; rho_off parameter; ABS_ON output; lambda2_th parameter
